simulink model "BierPong_dotz__00"  (R2021a)
settings: Solver=VariableStepAuto  StartTime=0.0  StopTime=10.0  RelTol=1e-3
model workspace (MAT data in the model file):
  c_w = 0.47
  d_Ball = 0.04
  d_cup = 0.095
  g = 9.81
  len = 2.1
  m_Ball = 2.7
  roh = 1.2
  s_cup = 0.05
libraries: simulink x1
settings Model: OrderedModelArguments=off  Creator=Max  LastModifiedBy=Max

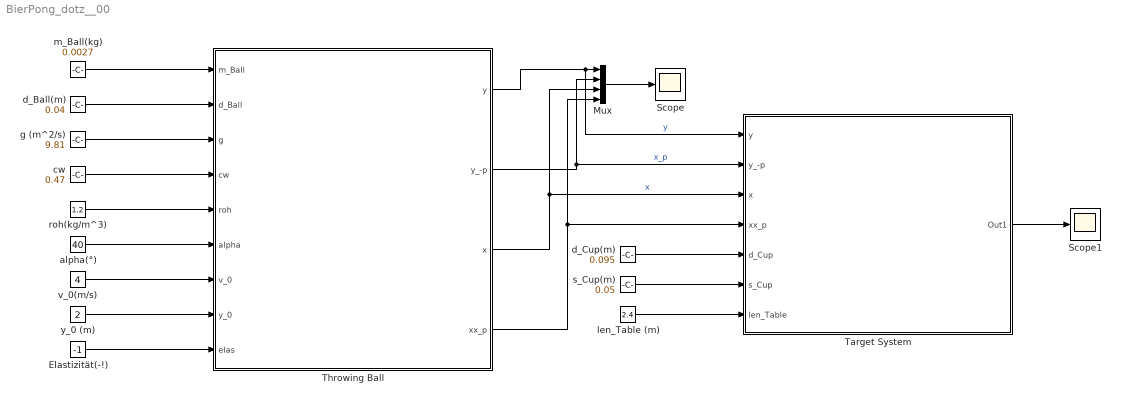
== system BierPong_dotz__00 ==
  Elastizität(-!) : Constant  Value=-1
  Mux : Mux
  Scope : Scope
  Scope1 : Scope
  Target System : Subsystem
  Throwing Ball : Subsystem
  alpha(°) : Constant  Value=40
  cw : Constant  Value=0.47
  d_Ball(m) : Constant  Value=0.04
  d_Cup(m) : Constant  Value=0.095
  g (m^2/s) : Constant  Value=9.81
  len_Table (m) : Constant  Value=2.4
  m_Ball(kg) : Constant  Value=0.0027
  roh(kg/m^3) : Constant  Value=1.2
  s_Cup(m) : Constant  Value=0.05
  v_0(m/s) : Constant  Value=4
  y_0 (m) : Constant  Value=2
  wires:
  m_Ball(kg)/1 -> Throwing Ball/1(m_Ball)
  d_Ball(m)/1 -> Throwing Ball/2(d_Ball)
  roh(kg/m^3)/1 -> Throwing Ball/5(roh)
  cw/1 -> Throwing Ball/4(cw)
  g (m^2/s)/1 -> Throwing Ball/3(g)
  Throwing Ball/1(y) -> Target System/1(y), Mux/1  "y"
  Throwing Ball/2(y_-p) -> Mux/2, Target System/2(y_-p)  "x_p"
  Throwing Ball/3(x) -> Mux/3, Target System/3(x)  "x"
  Throwing Ball/4(xx_p) -> Target System/4(xx_p), Mux/4
  Mux/1 -> Scope/1
  alpha(°)/1 -> Throwing Ball/6(alpha)
  v_0(m/s)/1 -> Throwing Ball/7(v_0)
  y_0 (m)/1 -> Throwing Ball/8(y_0)
  len_Table (m)/1 -> Target System/7(len_Table)
  s_Cup(m)/1 -> Target System/6(s_Cup)
  d_Cup(m)/1 -> Target System/5(d_Cup)
  Elastizität(-!)/1 -> Throwing Ball/9(elas)
  Target System/1(Out1) -> Scope1/1

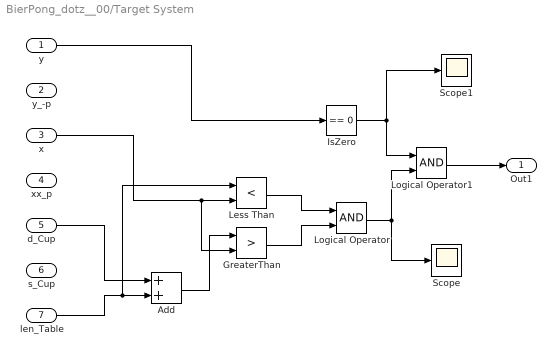
== system BierPong_dotz__00/Target System ==
  y : Inport
  y_-p : Inport  Port=2
  x : Inport  Port=3
  xx_p : Inport  Port=4
  d_Cup : Inport  Port=5
  s_Cup : Inport  Port=6
  len_Table : Inport  Port=7
  Add : Sum
  GreaterThan : RelationalOperator  Operator=>  OutDataTypeStr=boolean  RndMeth=Simplest
  IsZero : simulink/Logic and Bit Operations/Compare To Zero  relop===  OutDataTypeStr=boolean
  Less Than : RelationalOperator  Operator=<  OutDataTypeStr=boolean  RndMeth=Simplest
  Logical Operator : Logic  AllPortsSameDT=off  OutDataTypeStr=boolean
  Logical Operator1 : Logic  AllPortsSameDT=off  OutDataTypeStr=boolean
  Scope : Scope
  Scope1 : Scope
  Out1 : Outport
  wires:
  d_Cup/1 -> Add/1
  len_Table/1 -> Less Than/1, Add/2
  Add/1 -> GreaterThan/1
  x/1 -> GreaterThan/2, Less Than/2
  GreaterThan/1 -> Logical Operator/2
  Less Than/1 -> Logical Operator/1
  y/1 -> IsZero/1
  Logical Operator/1 -> Logical Operator1/2, Scope/1
  IsZero/1 -> Logical Operator1/1, Scope1/1
  Logical Operator1/1 -> Out1/1

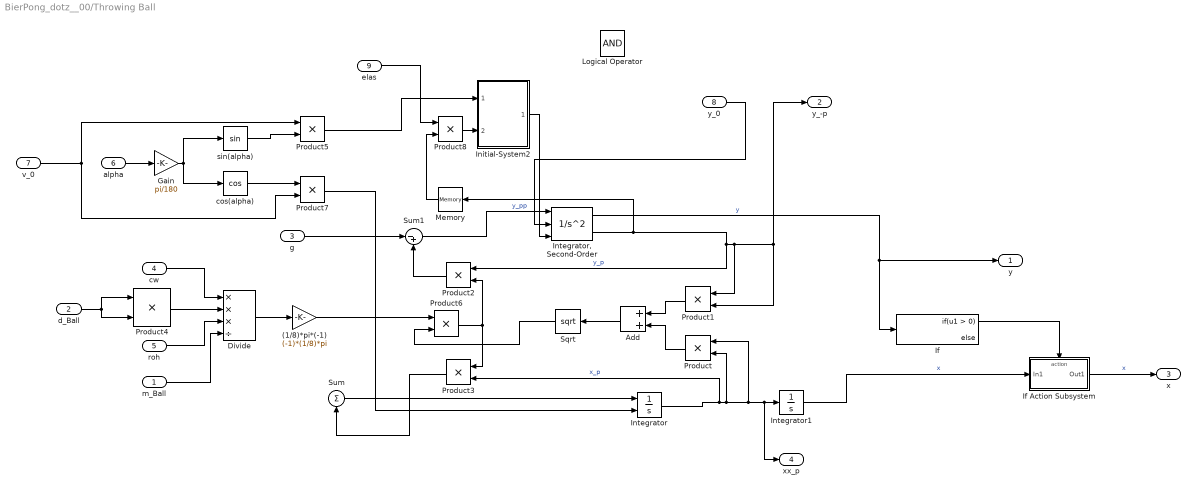
== system BierPong_dotz__00/Throwing Ball ==
  m_Ball : Inport
  d_Ball : Inport  Port=2
  g : Inport  Port=3
  cw : Inport  Port=4
  roh : Inport  Port=5
  alpha : Inport  Port=6
  v_0 : Inport  Port=7
  y_0 : Inport  Port=8
  elas : Inport  Port=9
  (1/8)*pi*(-1) : Gain  Gain=(-1)*(1/8)*pi
  Add : Sum
  Divide : Product  Inputs=***/
  Gain : Gain  Gain=pi/180
  If : If
  If Action Subsystem : Subsystem  TreatAsAtomicUnit=on
  Initial-System2 : Subsystem
  Integrator : Integrator  InitialConditionSource=external  InitialCondition=2
  "Integrator, Second-Order" : SecondOrderIntegrator  ICSourceX=external  LimitX=on  LowerLimitX=0.0  ICSourceDXDT=external  ReinitDXDTwhenXreachesSaturation=on
  Integrator1 : Integrator  LimitOutput=on  LowerSaturationLimit=0
  Logical Operator : Logic  AllPortsSameDT=off  OutDataTypeStr=boolean
  Memory : Memory
  Product{,1..8} (9 alike) : Product
  Sqrt : Sqrt  SaturateOnIntegerOverflow=on
  Sum : Sum  Inputs=|+
  Sum1 : Sum  Inputs=|-+
  cos(alpha) : Trigonometry  Operator=cos
  sin(alpha) : Trigonometry  OutputSignalType=real
  y : Outport
  y_-p : Outport  Port=2
  x : Outport  Port=3
  xx_p : Outport  Port=4
  wires:
  Product/1 -> Add/2
  "Integrator, Second-Order"/2 -> Memory/1, y_-p/1, Product1/2, Product1/1, Product2/1  "y_p"
  Product2/1 -> Sum1/2
  Integrator/1 -> Product3/2, Product/2, Product/1, xx_p/1, Integrator1/1  "x_p"
  Product3/1 -> Sum/1
  Sqrt/1 -> Product6/2
  Product1/1 -> Add/1
  Add/1 -> Sqrt/1
  Product6/1 -> Product2/2, Product3/1
  d_Ball/1 -> Product4/2, Product4/1
  cw/1 -> Divide/1
  Divide/1 -> (1/8)*pi*(-1)/1
  (1/8)*pi*(-1)/1 -> Product6/1
  g/1 -> Sum1/1
  Sum/1 -> Integrator/1
  Product4/1 -> Divide/2
  roh/1 -> Divide/3
  m_Ball/1 -> Divide/4
  Integrator1/1 -> If Action Subsystem/1(In1)  "x"
  "Integrator, Second-Order"/1 -> y/1, If/1  "y"
  If/1 -> If Action Subsystem/Action
  If Action Subsystem/1(Out1) -> x/1  "x"
  Gain/1 -> cos(alpha)/1, sin(alpha)/1
  v_0/1 -> Product7/2, Product5/1
  sin(alpha)/1 -> Product5/2
  cos(alpha)/1 -> Product7/1
  Product5/1 -> Initial-System2/1(Initial Value)
  Product7/1 -> Integrator/2
  y_0/1 -> "Integrator, Second-Order"/2
  alpha/1 -> Gain/1
  Sum1/1 -> "Integrator, Second-Order"/1  "y_pp"
  Initial-System2/1(OutBus) -> "Integrator, Second-Order"/3
  Product8/1 -> Initial-System2/2(Move Value)
  Memory/1 -> Product8/2
  elas/1 -> Product8/1

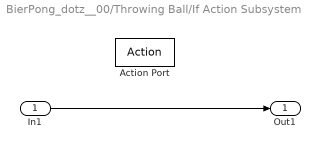
== system BierPong_dotz__00/Throwing Ball/If Action Subsystem ==
  In1 : Inport
  Action Port : ActionPort  ActionPortLabel=if(u1 > 0)
  Out1 : Outport
  wires:
  In1/1 -> Out1/1

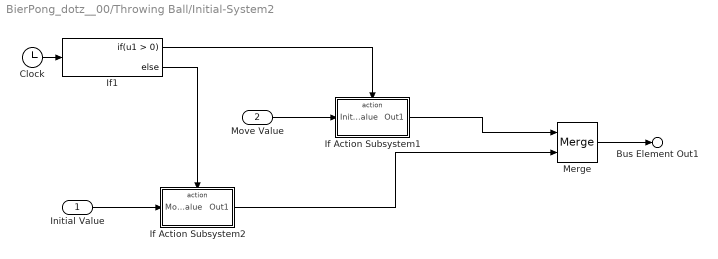
== system BierPong_dotz__00/Throwing Ball/Initial-System2 ==
  Initial Value : Inport
  Move Value : Inport  Port=2
  Clock : Clock
  If Action Subsystem1 : Subsystem  TreatAsAtomicUnit=on
  If Action Subsystem2 : Subsystem  TreatAsAtomicUnit=on
  If1 : If
  Merge : Merge
  Bus Element Out1 : Outport  PortName=OutBus  Element=signal1
  wires:
  If Action Subsystem1/1(Out1) -> Merge/1
  Merge/1 -> Bus Element Out1/1
  If1/1 -> If Action Subsystem1/Action
  If1/2 -> If Action Subsystem2/Action
  If Action Subsystem2/1(Out1) -> Merge/2
  Clock/1 -> If1/1
  Move Value/1 -> If Action Subsystem1/1(Initial Value)
  Initial Value/1 -> If Action Subsystem2/1(Move Value)

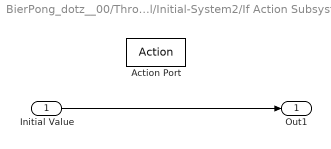
== system BierPong_dotz__00/Throwing Ball/Initial-System2/If Action Subsystem1 ==
  Initial Value : Inport
  Action Port : ActionPort  ActionPortLabel=if(u1 > 0)
  Out1 : Outport
  wires:
  Initial Value/1 -> Out1/1

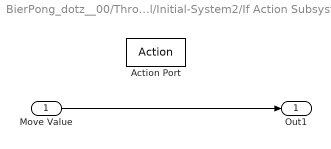
== system BierPong_dotz__00/Throwing Ball/Initial-System2/If Action Subsystem2 ==
  Move Value : Inport
  Action Port : ActionPort  ActionPortLabel=else
  Out1 : Outport
  wires:
  Move Value/1 -> Out1/1
